simulink model "animation"  (R2018a)
settings: Solver=VariableStepAuto  StartTime=0.0  StopTime=100000  MaxStep=0.2  RelTol=1e-3
PreLoadFcn:
  | param
libraries: simulink x3
settings Model: PacingRate=100  Creator=mark  LastModifiedBy=mark

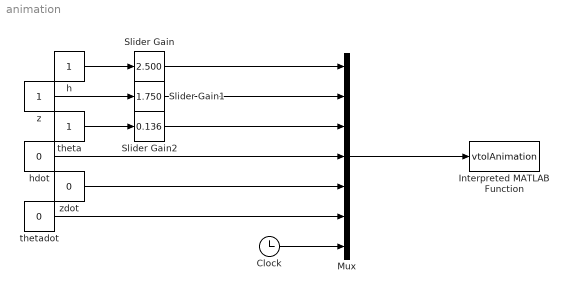
== system animation ==
  Clock : Clock
  Interpreted MATLAB Function : MATLABFcn  MATLABFcn=vtolAnimation  OutputDimensions=0
      mask help: VtolAnimation
  Mux : Mux  Inputs=7
  Slider Gain : simulink/Math Operations/Slider Gain  gain=2.500  low=0  high=5
  Slider Gain1 : simulink/Math Operations/Slider Gain  gain=1.750  low=0  high=5
  Slider Gain2 : simulink/Math Operations/Slider Gain  gain=0.136  low=-1.7  high=1.7
  h : Constant
  hdot : Constant  Value=0
  "theta " : Constant
  thetadot : Constant  Value=0
  z : Constant
  zdot : Constant  Value=0
  wires:
  Mux/1 -> Interpreted MATLAB Function/1
  Slider Gain/1 -> Mux/1
  Slider Gain1/1 -> Mux/2
  Slider Gain2/1 -> Mux/3
  h/1 -> Slider Gain/1
  z/1 -> Slider Gain1/1
  "theta "/1 -> Slider Gain2/1
  hdot/1 -> Mux/4
  zdot/1 -> Mux/5
  thetadot/1 -> Mux/6
  Clock/1 -> Mux/7
